simulink model "sl_groundvehicleDynamics"  (R2025a)
settings: Solver=ode45  StartTime=0.0  StopTime=1500  RelTol=1e-5  EnableMultiTasking=on
InitFcn:
  | mdl_robot;
undefined symbols (not defined in the file): robot, waypoints
libraries: simulink x4, mobileRoboticsLib x3, simulink_extras x2
settings Model: Creator=sriramn  LastModifiedBy=aidenkorbs
settings SolverCC: ZeroCrossAlgorithm=Adaptive  AlgebraicLoopSolver=TrustRegion
settings DataIOCC: LimitDataPoints=on  SaveFormat=Array  ReturnWorkspaceOutputs=off
settings OptimizationCC: ReuseModelBlockBuffer=off  LifeSpan=inf
settings DebuggingCC: SolverPrmCheckMsg=warning  UnconnectedInputMsg=warning  UnconnectedOutputMsg=warning  UnconnectedLineMsg=warning  AllowSymbolicDim=off  SFUnexpectedBacktrackingDiag=warning  SFNoUnconditionalDefaultTransitionDiag=warning  SFExecutionAtInitializationDiag=none  ArithmeticOperatorsInVariantConditions=warning
settings HardwareCC: ProdBitPerPointer=32.0  ProdBitPerSizeT=32.0  ProdBitPerPtrDiffT=32.0  ProdLargestAtomicFloat=None  ProdIntDivRoundTo=Undefined  ProdEndianess=Unspecified  ProdWordSize=32.0  ProdHWDeviceType=32-bit Generic
settings ModelReferenceCC: EnableRefExpFcnMdlSchedulingChecks=on  ModelReferenceMinAlgLoopOccurrences=on  PropagateSignalLabelsOutOfModel=off
settings SFSimCC: SimUseLocalCustomCode=off  CustomCodeUndefinedFunction=UseInterfaceOnly
settings RTWCC: RTWUseLocalCustomCode=off  GPUComputeCapability=3.5
settings CodeAppCC: StateflowObjectComments=on
settings GRTTargetCC: TargetLangStandard=C89/C90 (ANSI)
settings ConfigComp: CovMetricSettings=dw  CovSaveCumulativeToWorkspaceVar=on  CovSaveSingleToWorkspaceVar=on  CovExternalEMLEnable=off  CovSFcnEnable=off
settings SimscapeCC: SimscapeNormalizeSystem=off
settings ConfigurationSet: Description=SimMechanics 2G
settings ExplorerConfigSet: InternalSimMechanicsExplorerSettings="<ExplorerConfiguration><canonicalview>planar_xy</canonicalview><AnimationSetting><BasePlaybackSpeed>1.0</BasePlaybackSpeed><PlaybackSpeedFactor>1.0</PlaybackSpeedFactor></AnimationSetting><TilePanel><TileInfo><Tiles Columns=\"1\" Count=\"1\" Rows=\"1\"><Column Left=\"2\" Weight=\"1\"/><Column Left=\"1628\"/><Row Top=\"2\" Weight=\"1\"/><Row Top=\"1072\"/><Tile Height=\"1\" Width=\"1\" X=\"0\" Y=\"0\"/></Tiles></TileInfo><SceneInfo><SceneViewer><BGColor><R>0.60000002384185791</R><G>0.60000002384185791</G><B>0.60000002384185791</B></BGColor><Camera><Position><X>0.22951840878551699</X><Y>0.32651610611526627</Y><Z>-0.27215421354393321</Z></Position><Center><X>-0.15775714411666431</X><Y>-0.15462825985839526</Y><Z>0.065702552916005602</Z></Center><Up><X>-0.56030137557930915</X><Y>0.72817587161684794</Y><Z>0.39474329445726858</Z></Up><Left>-0.21481383955700509</Left><Right>0.21481383955700509</Right><Bottom>-0.27569784609469139</Bottom><Top>0.27569784609469139</Top></Camera></SceneViewer></SceneInfo></TilePanel></ExplorerConfiguration>"

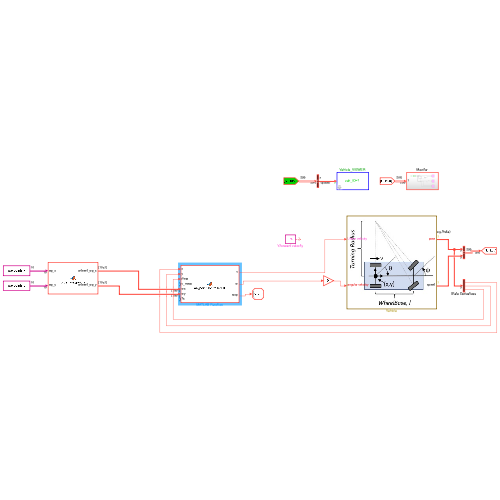
[thumbnail: Simulink's stored preview of the top-level diagram]
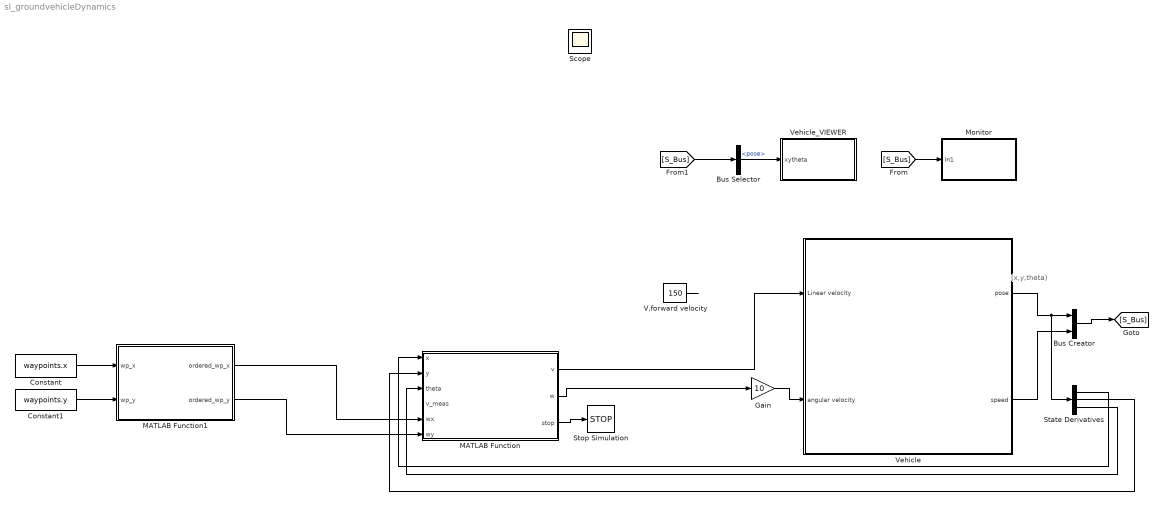
== system sl_groundvehicleDynamics ==
  note: (x,y,theta)
  Bus Creator : BusCreator  Inputs=2
  Bus Selector : BusSelector  OutputSignals=pose
  Constant : Constant  Value=waypoints.x
  Constant1 : Constant  Value=waypoints.y
  Gain : Gain  Gain=10
  MATLAB Function : MATLAB Function  TreatAsAtomicUnit=on
  MATLAB Function1 : MATLAB Function  TreatAsAtomicUnit=on
  Monitor : Subsystem
  State Derivatives : Demux  Outputs=3
  Stop Simulation : Stop
  V,forward velocity : Constant  Value=150
  Vehicle : Subsystem
      mask Display: image('vehicle.jpg');
  Vehicle_VIEWER : Subsystem  mask{wp_mat=[waypoints.x(:), waypoints.y(:)], veh_ID_num=1, veh_init_xytheta=[robot.X robot.Y robot.Theta], Ts=0.5}
      mask prompts: wp_mat "Waypoint matrix for arena [x_col, y_col] (m)"; veh_ID_num "Vehicle ID number"; veh_init_xytheta "Initial pose [x,y,theta]"; Ts "Sample time for updating animation (secs)"
      mask TypeOptions veh_ID_num: 1 | 2 | 3 | 4
      mask DialogControl Control2 Prompt: Animate simulation of Differential Drive Robot (DDR)
      mask Display: fprintf('veh_ID=%d',veh_ID_num);
  Scope : Scope
      settings: ActiveDisplayYMinimum=0.07  ActiveDisplayYMaximum=0.09
  wires:
  [S_Bus] -> Monitor/1(In1)
  [S_Bus] -> Bus Selector/1
  Vehicle/1(pose) -> State Derivatives/1, Bus Creator/1
  Vehicle/2(speed) -> Bus Creator/2
  Bus Creator/1 -> [S_Bus]
  Bus Selector/1 -> Vehicle_VIEWER/1(xytheta)  "<pose>"
  MATLAB Function/2(w) -> Gain/1
  V,forward velocity/1 -> ?
  State Derivatives/3 -> MATLAB Function/3(theta)
  Gain/1 -> Vehicle/2(angular velocity)
  State Derivatives/2 -> MATLAB Function/2(y)
  State Derivatives/1 -> MATLAB Function/1(x)
  MATLAB Function/3(stop) -> Stop Simulation/1
  Constant/1 -> MATLAB Function1/1(wp_x)
  Constant1/1 -> MATLAB Function1/2(wp_y)
  MATLAB Function1/1(ordered_wp_x) -> MATLAB Function/5(wx)
  MATLAB Function1/2(ordered_wp_y) -> MATLAB Function/6(wy)
  MATLAB Function/1(v) -> Vehicle/1(Linear velocity)

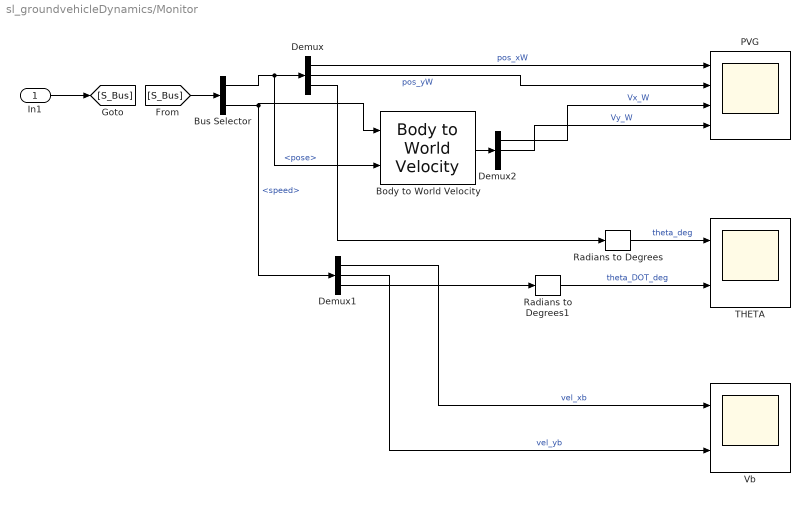
== system sl_groundvehicleDynamics/Monitor ==
  In1 : Inport
  Body to World Velocity : mobileRoboticsLib/Utilities/Body to World Velocity
      settings: SourceProductName=Mobile Robotics Simulation Toolbox
  Bus Selector : BusSelector  OutputSignals=pose,speed
  Demux : Demux  Outputs=3
  Demux1 : Demux  Outputs=3
  Demux2 : Demux  Outputs=3
  PVG : Scope  NumInputPorts=4
      settings: ActiveDisplayYMinimum=-3.02358  ActiveDisplayYMaximum=27.35477
  Radians to Degrees : simulink_extras/Transformations/Radians to Degrees
  Radians to Degrees1 : simulink_extras/Transformations/Radians to Degrees
  THETA : Scope  NumInputPorts=2
      settings: ActiveDisplayYMinimum=-8.72937  ActiveDisplayYMaximum=60.06611  DataLoggingVariableName=ScopeData2
  Vb : Scope  NumInputPorts=2
      settings: ActiveDisplayYMinimum=0.05577  ActiveDisplayYMaximum=0.8929
  wires:
  In1/1 -> [S_Bus]
  [S_Bus] -> Bus Selector/1
  Demux/1 -> PVG/1  "pos_xW"
  Demux/2 -> PVG/2  "pos_yW"
  Radians to Degrees1/1 -> THETA/2  "theta_DOT_deg"
  Radians to Degrees/1 -> THETA/1  "theta_deg"
  Demux1/3 -> Radians to Degrees1/1
  Demux/3 -> Radians to Degrees/1
  Bus Selector/1 -> Body to World Velocity/2, Demux/1  "<pose>"
  Bus Selector/2 -> Demux1/1, Body to World Velocity/1  "<speed>"
  Body to World Velocity/1 -> Demux2/1
  Demux2/1 -> PVG/3  "Vx_W"
  Demux2/2 -> PVG/4  "Vy_W"
  Demux1/1 -> Vb/1  "vel_xb"
  Demux1/2 -> Vb/2  "vel_yb"

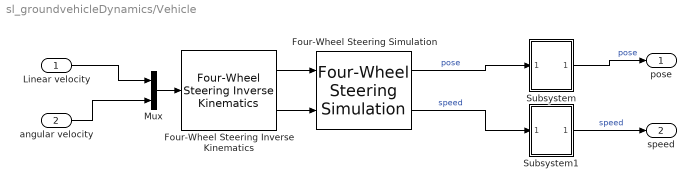
== system sl_groundvehicleDynamics/Vehicle ==
  Linear velocity : Inport
  angular velocity : Inport  Port=2
  Four-Wheel Steering Inverse Kinematics : mobileRoboticsLib/Kinematic Models/Four-Wheel Steering/Four-Wheel Steering Inverse Kinematics  wheelRadius=0.1  frontWheelDist=0.25  rearWheelDist=0.25  ikMode=Front Steering
      settings: SourceProductName=Mobile Robotics Simulation Toolbox
  Four-Wheel Steering Simulation : mobileRoboticsLib/Kinematic Models/Four-Wheel Steering/Four-Wheel Steering Simulation  wheelRadius=0.1  frontWheelDist=0.25  rearWheelDist=0.25  initX=robot.X  initY=robot.Y  initAngle=robot.Theta  Ts=0.05
      settings: SourceProductName=Mobile Robotics Simulation Toolbox
  Mux : Mux  Inputs=2
  Subsystem : Subsystem
  Subsystem1 : Subsystem
  pose : Outport  VectorParamsAs1DForOutWhenUnconnected=off
  speed : Outport  Port=2
  wires:
  angular velocity/1 -> Mux/2
  Linear velocity/1 -> Mux/1
  Mux/1 -> Four-Wheel Steering Inverse Kinematics/1
  Four-Wheel Steering Simulation/1 -> Subsystem/1(In1)  "pose"
  Four-Wheel Steering Simulation/2 -> Subsystem1/1(In1)  "speed"
  Four-Wheel Steering Inverse Kinematics/1 -> Four-Wheel Steering Simulation/1
  Four-Wheel Steering Inverse Kinematics/2 -> Four-Wheel Steering Simulation/2
  Subsystem/1(pose) -> pose/1  "pose"
  Subsystem1/1(speed) -> speed/1  "speed"

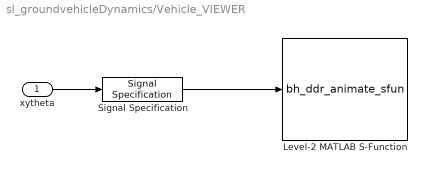
== system sl_groundvehicleDynamics/Vehicle_VIEWER ==
  xytheta : Inport
  Level-2 MATLAB S-Function : M-S-Function  FunctionName=bh_ddr_animate_sfun  Parameters=Ts, wp_mat, veh_ID_num, veh_init_xytheta
  Signal Specification : SignalSpecification  Dimensions=3
  wires:
  xytheta/1 -> Signal Specification/1
  Signal Specification/1 -> Level-2 MATLAB S-Function/1

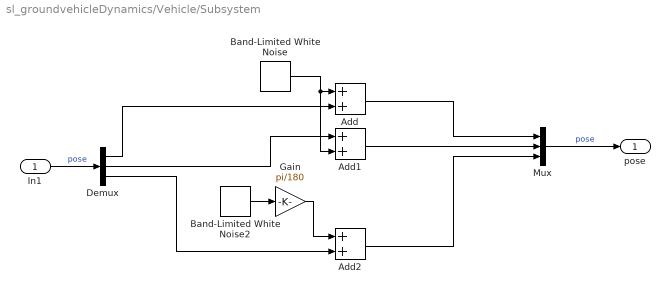
== system sl_groundvehicleDynamics/Vehicle/Subsystem ==
  In1 : Inport
  Add : Sum
  Add1 : Sum
  Add2 : Sum
  Band-Limited White Noise : simulink/Sources/Band-Limited White Noise  Cov=[0.001]  Ts=0.1  seed=[23341]
  Band-Limited White Noise2 : simulink/Sources/Band-Limited White Noise  Cov=[0.41]  Ts=0.1  seed=[23341]
  Demux : Demux  Outputs=3
  Gain : Gain  Gain=pi/180
  Mux : Mux  Inputs=3
  pose : Outport
  wires:
  Add1/1 -> Mux/2
  Add2/1 -> Mux/3
  Demux/2 -> Add1/1
  Band-Limited White Noise2/1 -> Gain/1
  Demux/3 -> Add2/2
  Band-Limited White Noise/1 -> Add1/2, Add/1
  In1/1 -> Demux/1  "pose"
  Demux/1 -> Add/2
  Gain/1 -> Add2/1
  Mux/1 -> pose/1  "pose"
  Add/1 -> Mux/1

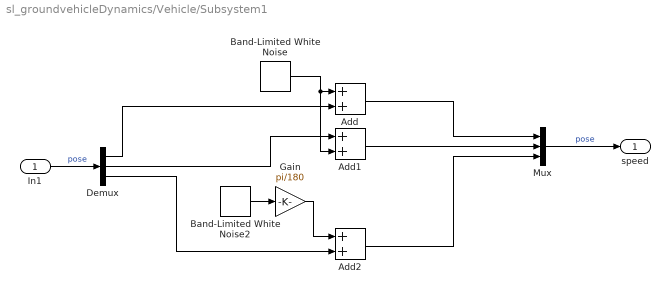
== system sl_groundvehicleDynamics/Vehicle/Subsystem1 ==
  In1 : Inport
  Add : Sum
  Add1 : Sum
  Add2 : Sum
  Band-Limited White Noise : simulink/Sources/Band-Limited White Noise  Cov=[0.001]  Ts=0.1  seed=[23341]
  Band-Limited White Noise2 : simulink/Sources/Band-Limited White Noise  Cov=[0.41]  Ts=0.1  seed=[23341]
  Demux : Demux  Outputs=3
  Gain : Gain  Gain=pi/180
  Mux : Mux  Inputs=3
  speed : Outport
  wires:
  Add1/1 -> Mux/2
  Add2/1 -> Mux/3
  Demux/2 -> Add1/1
  Band-Limited White Noise2/1 -> Gain/1
  Demux/3 -> Add2/2
  Band-Limited White Noise/1 -> Add1/2, Add/1
  In1/1 -> Demux/1  "pose"
  Demux/1 -> Add/2
  Gain/1 -> Add2/1
  Mux/1 -> speed/1  "pose"
  Add/1 -> Mux/1

== matlab function sl_groundvehicleDynamics/MATLAB Function1 ==
  data: wp_x input; ordered_wp_x output; ordered_wp_y output; wp_y input
function [ordered_wp_x, ordered_wp_y]= order_waypoints(wp_x, wp_y)
    % organise the waypoints in the way the function expects
    waypoints = [wp_x(:), wp_y(:)];
    num_waypoints = size(waypoints, 1);

    % set up waypoint index array and empty route array
    waypoint_idx = 1:num_waypoints;
    route = zeros(1, num_waypoints);
    
    % set the starting point as the first waypoint in the list
    route(1) = 1;
    waypoint_idx(1) = [];

    %% nearest neighbour
    % nearest neighbour loop
    for i = 1:num_waypoints-1
        % compute distances to all remaining waypoints
        current_waypoint = waypoints(route(i), :);
        distances = zeros(1, length(waypoint_idx));
        for j = 1:length(waypoint_idx)
            next_potential_point = waypoints(waypoint_idx(j), :);
            distances(j) = pdist2(current_waypoint, next_potential_point);
        end
        % select closest point to travel to next
        [~, min_idx] = min(distances);
        route(i+1) = waypoint_idx(min_idx);
        waypoint_idx(min_idx) = [];
    
    end

    %% 2-opt swap
    % optimise n-n generated route with 2-opt swap
    improved = true;
    tolerance = 1e-12;
    
    % helper method for computing distance
    get_dist = @(a,b) pdist2(waypoints(a, :), waypoints(b, :));
    
    % compute original length of n-n generated route
    len_before = 0;
    for i=1:num_waypoints-1
        len_before = len_before + pdist2(waypoints(route(i), :), waypoints(route(i+1), :));
    end
    %disp("Total length of n-n generated route: " + len_before);
    
    num_iterations = 0;
    while improved
        num_iterations = num_iterations + 1;
        improved = false;
        for i = 1:num_waypoints-3
            a = route(i);
            b = route(i+1);
            for j = i+2:num_waypoints-1
                c = route(j);
                d = route(j+1);
                
                % swap if it makes the route shorter
                delta = (get_dist(a,c) + get_dist(b,d)) - (get_dist(a,b) + get_dist(c,d));
                if delta < -tolerance
                    route(i+1:j) = route(j:-1:i+1);
                    improved = true;
                end
            end
        end
    end
    
    len_after = 0;
    for i=1:num_waypoints-1
        len_after = len_after + pdist2(waypoints(route(i), :), waypoints(route(i+1), :));
    end
    %disp("Total length of 2-opt swap optimised route: " + len_after);
    
    %disp("Total number of 2-opt swap iterations: " + num_iterations);

    %% return the ordered waypoint vectors
    ordered_wp_x = waypoints(route, 1);
    ordered_wp_y = waypoints(route, 2);

end

== matlab function sl_groundvehicleDynamics/MATLAB Function ==
  data: v output; x input; w output; y input; theta input; v_meas input; wx input; wy input; stop output
function [v, w, stop] = waypointControllerPID(x, y, theta, v_meas, wx, wy)
%% Tuning Variables
% Controller sample time (s) – set to your model's controller step
Ts = 0.02;

% Heading PID (for w)
Kp_h = 1.6;     Ki_h = 0.20;   Kd_h = 0.05;
w_max = 1.2;                  % [rad/s] limit
i_lim_h = 2.0;                % integral clamp

% Speed PI (for v)
Kp_v = 1.0;     Ki_v = 0.5;
v_max = 100;   v_min = 0.0;   % [m/s]
i_lim_v = 5.0;

% Waypoint logic
capture_R   = 5.0;            % [m] switch waypoint
slow_R      = 40.0;           % [m] start slowing down near wp
e_slow_max  = pi/2;           % slow for big heading error (≈90°)

% Cruise bias (regular speed)
v_cruise    = 20;            % [m/s]
%% 

wx = wx(:);
wy = wy(:);
N  = numel(wx);

% Persistent state
persistent idx ih iv eh_prev Nprev
if isempty(idx);     idx = 1;        end
if isempty(ih);      ih  = 0.0;      end
if isempty(iv);      iv  = 0.0;      end
if isempty(eh_prev); eh_prev = 0.0;  end
if isempty(Nprev);   Nprev = N;      end

% Reset index if waypoint list size changed or index out of range
if (N ~= Nprev) || (idx < 1) || (idx > max(N,1))
    idx = 1;
    ih = 0.0; iv = 0.0; eh_prev = 0.0;
    Nprev = N;
end

% Default outputs
v = 0.0; w = 0.0; stop = 0;

% Guard empty waypoint list
if N == 0
    stop = 1;
    return;
end

% Current target waypoint
xw = wx(idx);  yw = wy(idx);

% Heading error (wrapped)
alpha = atan2(yw - y, xw - x);
eh    = wrapErr(alpha - theta);     % [-pi, pi]

% Distance to waypoint
d = hypot(x - xw, y - yw);

% --------- Speed scheduling (feedforward target) ----------
% Slow for big heading error
slow_heading   = clamp(1.0 - abs(eh)/e_slow_max, 0.0, 1.0);
% Slow as you approach the waypoint
slow_distance  = clamp(d/slow_R, 0.0, 1.0);
% Base desired speed
v_des = v_cruise * slow_heading * slow_distance;
v_des = clamp(v_des, v_min, v_max);

% --------- Heading PID -> angular rate w ------------------
ih = clamp(ih + eh*Ts, -i_lim_h, i_lim_h);    % integral
de = (eh - eh_prev) / max(Ts, 1e-6);          % derivative
w  = Kp_h*eh + Ki_h*ih + Kd_h*de;
w  = clamp(w, -w_max, w_max);
eh_prev = eh;

% --------- Speed PI -> forward speed v --------------------
ev = v_des - v_meas;
iv = clamp(iv + ev*Ts, -i_lim_v, i_lim_v);
v  = v_meas + Kp_v*ev + Ki_v*iv;              % absolute speed cmd
v  = clamp(v, v_min, v_max);

% --------- Waypoint switching & stop ----------------------
if d < capture_R
    if idx < N
        idx = idx + 1;
        % optional: clear heading integrator on wp switch
        ih = 0.0;
    else
        v = 0.0; w = 0.0;
        stop = 1;
    end
end

end

% ===== helpers =====
function z = clamp(x, a, b)
    z = min(max(x, a), b);
end

function e = wrapErr(x)
    % wrap to [-pi, pi]
    e = atan2(sin(x), cos(x));
end
